simulink model "MIL4L3_SW6_V1_20220211"  (R2018b)
(part 32 of 52)

  Gain218/1 -> Data Type Conversion224/1, IMAPva_d_obj_status/1  "IMAPva_d_obj_status"
  Gain318/1 -> Data Type Conversion32/1, IMAPve_d_BCM_LowBeam_State/1
  SDFAva_g_obj_length/1 -> Gain214/1
  Gain67/1 -> Data Type Conversion96/1, IMAPve_d_TCU_AT_Failure/1
  Gain62/1 -> Data Type Conversion126/1, IMAPve_g_ESC_RR_WhlSpd/1
  Gain325/1 -> Data Type Conversion349/1, IMAPve_d_TBOX_LocalTimeS/1
  Gain63/1 -> Data Type Conversion127/1, IMAPve_d_ESC_FL_Wheel_Pulse/1
  Gain11/1 -> Data Type Conversion149/1, IMAPva_g_ORI_Obj_Width/1  "IMAPva_g_ORI_Obj_Width"
  Gain375/1 -> Data Type Conversion484/1, IMAPve_g_ORI_R1_Dxstart/1  "IMAPve_g_ORI_R1_Dxstart"
  ? -> Gain361/1
  Gain57/1 -> Data Type Conversion121/1, IMAPve_d_ESC_RL_WheelPulVal/1
  Data Type Conversion175/1 -> Terminator166/1  "ob_IMAPve_g_ORI_R0_C2"
  ? -> Gain369/1
  Data Type Conversion343/1 -> Terminator348/1  "ob_IMAPve_d_TBOX_LocalTimeM"
  Gain166/1 -> Data Type Conversion251/1, IMAPve_g_R0_C2/1  "IMAPve_g_R0_C2"
  Gain61/1 -> Data Type Conversion125/1, IMAPve_g_ESC_RL_WhlSpd/1
  Gain250/1 -> Data Type Conversion180/1, IMAPve_g_ORI_R0_VR/1  "IMAPve_g_ORI_R0_VR"
  Gain409/1 -> Data Type Conversion428/1, IMAPva_g_ORI_Obj_LAngleStdDev/1  "IMAPva_g_ORI_Obj_LAngleStdDev"
  Gain216/1 -> Data Type Conversion222/1, IMAPva_d_obj_class/1  "IMAPva_d_obj_class"
  Gain406/1 -> Data Type Conversion437/1, IMAPva_g_ORI_Obj_HeadingStdDev/1  "IMAPva_g_ORI_Obj_HeadingStdDev"
  Gain41/1 -> Data Type Conversion53/1, IMAPve_d_ACU_Driver_Belt/1
  Gain54/1 -> Data Type Conversion118/1, IMAPve_d_ESC_ABS_Active/1
  Gain60/1 -> Data Type Conversion124/1, IMAPve_g_ESC_FR_WhlSpd/1
  Gain211/1 -> Data Type Conversion413/1, IMAPve_d_MP5_APA_ModeSelect/1
  Data Type Conversion113/1 -> Terminator105/1  "ob_IMAPve_d_ESC_ESC_Active"
  Gain58/1 -> Data Type Conversion122/1, IMAPve_d_ESC_RR_WheelPulVal/1
  Gain441/1 -> IMAPve_d_ORI_FS_Fog/1, Data Type Conversion335/1  "IMAPve_d_ORI_FS_Fog"
  Data Type Conversion398/1 -> Terminator394/1  "ob_IMAPva_g_ORI_Obj_RelVelStdDev"
  SDFAve_g_ORI_L1_C1/1 -> Gain266/1
  Data Type Conversion194/1 -> Terminator185/1  "ob_IMAPve_d_LF_Radar_Status"
  Data Type Conversion318/1 -> Terminator309/1  "ob_IMAPve_d_MP5_DMS_UserAccount"
  Gain6/1 -> IMAPva_g_ORI_Obj_RelVel/1, Data Type Conversion144/1  "IMAPva_g_ORI_Obj_RelVel"
  Data Type Conversion250/1 -> Terminator241/1  "ob_IMAPve_g_R0_C1"
  Data Type Conversion170/1 -> Terminator161/1  "ob_IMAPve_g_ORI_L1_VR"
  Gain56/1 -> Data Type Conversion120/1, IMAPve_d_ESC_FR_WheelPulVal/1
  SDFAve_g_L1_VIEW_RANGE/1 -> Gain161/1
  Gain184/1 -> Data Type Conversion36/1, IMAPve_d_AEB_Switch/1
  Gain369/1 -> Data Type Conversion477/1, IMAPve_g_ORI_RoadedgeR0_C3/1  "IMAPve_g_ORI_RoadedgeR0_C3"
  Data Type Conversion253/1 -> Terminator244/1  "ob_IMAPve_g_R0_VR"
  SDFAve_g_ORI_R1_C0/1 -> Gain239/1
  Gain223/1 -> Data Type Conversion211/1, IMAPva_g_obj_acc_x/1  "IMAPva_g_obj_acc_x"
  SDFAve_g_R0_C3_BACK_COEF/1 -> Gain137/1
  Gain69/1 -> Data Type Conversion98/1, IMAPve_d_TCU_Gear_Engage/1
  Gain80/1 -> Data Type Conversion56/1, IMAPve_d_BCM_BrakeLamp_State/1
  Data Type Conversion157/1 -> Terminator148/1  "ob_IMAPve_g_ORI_L0_C0"
  Data Type Conversion211/1 -> Terminator202/1  "ob_IMAPva_g_obj_acc_x"
  ? -> Gain398/1
  Data Type Conversion283/1 -> Terminator274/1  "ob_IMAPve_g_L0_C1_Back"
  Gain230/1 -> Data Type Conversion195/1, IMAPve_d_RF_Radar_Status/1  "IMAPve_d_RF_Radar_Status"
  ? -> Gain358/1
  Gain44/1 -> Data Type Conversion88/1, IMAPve_d_TCU_Actual_Gear/1
  ? -> Gain375/1
  Gain52/1 -> Data Type Conversion116/1, IMAPve_d_ESC_VehSpd_Valid/1
  Data Type Conversion272/1 -> Terminator263/1  "ob_IMAPve_g_R1_C1"
  SDFAve_d_sen_sta_RF_radar/1 -> Gain230/1
  Gain109/1 -> Data Type Conversion201/1, IMAPve_d_TSR_Sign_Type/1  "IMAPve_d_TSR_Sign_Type"
  Data Type Conversion353/1 -> Terminator356/1  "ob_IMAPve_d_Outside_Temp"
  Gain143/1 -> Data Type Conversion282/1, IMAPve_g_L0_C0_Back/1  "IMAPve_g_L0_C0_Back"
  Gain55/1 -> Data Type Conversion119/1, IMAPve_d_ESC_FL_WheelPulVal/1
  Gain448/1 -> IMAPve_d_JA_Alert_Switch/1, Data Type Conversion24/1
  ? -> Gain377/1
  Gain33/1 -> Data Type Conversion81/1, IMAPve_g_EMS_MinTWhl/1
  Gain426/1 -> Data Type Conversion396/1, IMAPva_g_ORI_Obj_AbsAxStdDev/1  "IMAPva_g_ORI_Obj_AbsAxStdDev"
  Gain46/1 -> Data Type Conversion111/1, IMAPve_d_ESC_OFF/1
  Gain72/1 -> Data Type Conversion90/1, IMAPve_d_EMS_Gearbox_CtlAvail/1
  SWINve_y_MP5_DMS_SmokingMonitor/1 -> Gain301/1
  Gain144/1 -> Data Type Conversion283/1, IMAPve_g_L0_C1_Back/1  "IMAPve_g_L0_C1_Back"
  Data Type Conversion196/1 -> Terminator187/1  "ob_IMAPve_d_LR_Radar_Status"
  Gain145/1 -> Data Type Conversion284/1, IMAPve_g_L0_C2_Back/1  "IMAPve_g_L0_C2_Back"
  Gain32/1 -> Data Type Conversion80/1, IMAPve_g_EMS_MaxTWhl_Offset/1
  SDFAva_y_obj_class/1 -> Gain216/1
  Data Type Conversion421/1 -> Terminator402/1  "ob_IMAPva_g_ORI_Obj_ExistProb"
  Gain295/1 -> Data Type Conversion218/1, IMAPve_d_MP5_DMS_DelUserNum/1  "IMAPve_d_MP5_DMS_DelUserNum"
  Gain37/1 -> Data Type Conversion109/1, IMAPve_d_ESC_Brake_Effort/1
  SDFAve_g_L1_C2_BACK_COEF/1 -> Gain120/1
  Gain416/1 -> Data Type Conversion421/1, IMAPva_g_ORI_Obj_ExistProb/1  "IMAPva_g_ORI_Obj_ExistProb"
  Data Type Conversion67/1 -> Terminator58/1  "ob_IMAPve_d_SAS_Clb_State"
  Data Type Conversion122/1 -> Terminator114/1  "ob_IMAPve_d_ESC_RR_WheelPulVal"
  Gain39/1 -> Data Type Conversion110/1, IMAPve_d_ESC_Veh_Standstill/1
  Data Type Conversion221/1 -> Terminator212/1  "ob_IMAPve_d_MP5_DMS_Sensity"
  Gain432/1 -> IMAPva_g_ORI_Obj_AbsAy/1, Data Type Conversion393/1  "IMAPva_g_ORI_Obj_AbsAy"
  SDFAve_g_L1_BACK_RANGE/1 -> Gain122/1
  SDFAva_y_obj_MotionStatus/1 -> Gain206/1
  SWINve_y_MP5_DMS_SideViewMonitor/1 -> Gain299/1
  Gain35/1 -> Data Type Conversion77/1, IMAPve_g_EMS_Pot_WhlT_Min/1
  Gain246/1 -> Data Type Conversion176/1, IMAPve_g_ORI_R0_C1/1  "IMAPve_g_ORI_R0_C1"
  Data Type Conversion286/1 -> Terminator277/1  "ob_IMAPve_g_L0_Range_Back"
  Data Type Conversion344/1 -> Terminator349/1  "ob_IMAPve_d_TBOX_LocalTimeD"
  SWINve_y_MP5_DMS_UsingPhoneMonitor/1 -> Gain300/1
  ? -> Gain417/1
  Data Type Conversion204/1 -> Terminator195/1  "ob_IMAPve_d_Camera_Status"
  Data Type Conversion189/1 -> Terminator180/1  "ob_IMAPve_d_ORI_R1_LT"
  Gain42/1 -> array_transfer10/2(Left_Light), Data Type Conversion50/1, IMAPve_d_BCM_Left_Light/1
  ? -> Gain373/1
  Gain103/1 -> IMAPve_d_Camera_Status/1, Data Type Conversion204/1  "IMAPve_d_Camera_Status"
  Gain20/1 -> Data Type Conversion103/1, IMAPve_g_ESC_VehSpd/1
  Gain136/1 -> Data Type Conversion293/1, IMAPve_g_R0_C2_Back/1  "IMAPve_g_R0_C2_Back"
  Gain436/1 -> IMAPve_d_ORI_FS_FrozenWindshield0/1, Data Type Conversion389/1  "IMAPve_d_ORI_FS_FrozenWindshield0"
  Data Type Conversion406/1 -> Terminator335/1  "ob_IMAPve_d_BCM_LeftTurn_Switch"
  SDFAve_g_R1_C2_COEF/1 -> Gain152/1
  Data Type Conversion244/1 -> Terminator235/1  "ob_IMAPve_d_L0_Type"
  SDFAve_g_ORI_R1_VR/1 -> Gain242/1
  Gain238/1 -> Data Type Conversion186/1, IMAPve_g_ORI_R1_C1/1  "IMAPve_g_ORI_R1_C1"
  Gain262/1 -> Data Type Conversion162/1, IMAPve_g_ORI_L0_W/1  "IMAPve_g_ORI_L0_W"
  Data Type Conversion70/1 -> Terminator61/1  "ob_IMAPve_g_SW_Angle"
  SDFAve_y_R0_DETECT_QUALITY/1 -> Gain169/1
  Gain30/1 -> Data Type Conversion76/1, IMAPve_g_EMS_Pot_WhlT_Max/1
  Gain12/1 -> Data Type Conversion150/1, IMAPva_d_ORI_Obj_ID/1  "IMAPva_d_ORI_Obj_ID"
  Data Type Conversion249/1 -> Terminator240/1  "ob_IMAPve_g_R0_C0"
  Gain312/1 -> Data Type Conversion21/1, IMAPve_d_RCTA_Swtich/1
  Gain26/1 -> Data Type Conversion108/1, IMAPve_g_ESC_DySlope/1
  Data Type Conversion465/1 -> Terminator446/1  "ob_IMAPve_g_ORI_RoadedgeL0_DxEnd"
  ? -> Gain414/1
  Data Type Conversion42/1 -> Terminator33/1  "ob_IMAPve_d_BCM_Opening_State"
  Gain29/1 -> Data Type Conversion75/1, IMAPve_d_EMS_ACC_Status/1
  Data Type Conversion367/1 -> Terminator365/1  "ob_IMAPve_d_ESC_LatAcc_Valid"
  SWINve_y_MP5_DMS_DeleteUserNum/1 -> Gain295/1
  Data Type Conversion452/1 -> Terminator433/1  "ob_IMAPve_g_ORI_L0_TypeConf"
  Data Type Conversion165/1 -> Terminator156/1  "ob_IMAPve_g_ORI_L1_C2"
  Data Type Conversion167/1 -> Terminator158/1  "ob_IMAPve_g_ORI_L1_C0"
  Gain38/1 -> Data Type Conversion87/1, IMAPve_g_EMS_Engine_Speed/1
  Data Type Conversion453/1 -> Terminator434/1  "ob_IMAPve_g_ORI_R0_TypeConf"
  Gain65/1 -> Data Type Conversion129/1, IMAPve_d_ESC_RL_Wheel_Pulse/1
  Gain269/1 -> IMAPve_g_ORI_L0_C2/1, Data Type Conversion155/1  "IMAPve_g_ORI_L0_C2"
  SDFAve_d_ORI_Obj_Num/1 -> Gain2/1
  Data Type Conversion129/1 -> Terminator116/1  "ob_IMAPve_d_ESC_RL_Wheel_Pulse"
  Gain423/1 -> Data Type Conversion399/1, IMAPva_g_ORI_Obj_RelVelyStdDev/1  "IMAPva_g_ORI_Obj_RelVelyStdDev"
  SDFAva_g_obj_vel_x/1 -> Gain221/1
  SDFAve_d_ORI_L1_Type/1 -> Gain255/1
  SDFAva_g_ORI_Obj_AbsAy/1 -> Gain432/1
  Gain17/1 -> Data Type Conversion100/1, IMAPve_g_ESC_LatAcc/1
  Data Type Conversion145/1 -> Terminator136/1  "ob_IMAPva_g_ORI_Obj_LongDis"
  Gain372/1 -> Data Type Conversion480/1, IMAPve_d_ORI_RoadedgeR0_Type/1  "IMAPve_d_ORI_RoadedgeR0_Type"
  Gain36/1 -> Data Type Conversion86/1, IMAPve_g_EMS_Driver_Torque/1
  Data Type Conversion371/1 -> Terminator369/1  "ob_IMAPve_d_ESC_ABS_AlarmSig"
  Gain174/1 -> Data Type Conversion241/1, IMAPve_g_L0_C3/1  "IMAPve_g_L0_C3"
  Gain73/1 -> Data Type Conversion131/1, IMAPve_d_ESC_Brake_Failsafe/1
  Gain287/1 -> Data Type Conversion61/1, IMAPve_d_Time_System_Clock/1
  Gain234/1 -> Data Type Conversion199/1, IMAPve_d_Fusion_Time_Stamp/1  "IMAPve_d_Fusion_Time_Stamp"
  Gain48/1 -> IMAPve_d_BCM_Right_Light/1, Data Type Conversion51/1, array_transfer10/3(Right_Light)
  Gain40/1 -> Data Type Conversion52/1, IMAPve_d_BCM_Ignition_State/1
  ? -> Gain406/1
  Data Type Conversion147/1 -> Terminator138/1  "ob_IMAPva_g_ORI_Obj_LAngle"
  SDFAve_g_L0_VIEW_RANGE/1 -> Gain175/1
  Data Type Conversion99/1 -> Terminator90/1  "ob_IMAPve_d_TCU_Select_ATMode"
  Data Type Conversion187/1 -> Terminator178/1  "ob_IMAPve_g_ORI_R1_C0"
  Gain25/1 -> Data Type Conversion107/1, IMAPve_g_ESC_DySlope_Accuracy/1
  Data Type Conversion43/1 -> Terminator34/1  "ob_IMAPve_d_BCM_Trunk_State"
  Gain177/1 -> Data Type Conversion244/1, IMAPve_d_L0_Type/1  "IMAPve_d_L0_Type"
  SDFAva_g_ORI_Obj_RelVely/1 -> Gain444/1
  SDFAve_y_Radar_State/1 -> Gain102/1
  Data Type Conversion148/1 -> Terminator139/1  "ob_IMAPva_g_ORI_Obj_RAngle"
  Data Type Conversion350/1 -> Terminator353/1  "ob_IMAPve_d_TBOX_LocalTime_Valid"
  Gain4/1 -> Data Type Conversion142/1, IMAPva_d_ORI_Obj_Class/1  "IMAPva_d_ORI_Obj_Class"
  Data Type Conversion144/1 -> Terminator135/1  "ob_IMAPva_g_ORI_Obj_RelVel"
  Gain222/1 -> Data Type Conversion210/1, IMAPva_g_obj_vel_y/1  "IMAPva_g_obj_vel_y"
  ? -> Gain374/1
  Data Type Conversion156/1 -> Terminator147/1  "ob_IMAPve_g_ORI_L0_C1"
  SDFAve_d_sen_sta_LB_radar/1 -> Gain231/1
  Data Type Conversion160/1 -> Terminator151/1  "ob_IMAPve_g_ORI_L0_VR"
  Gain400/1 -> Data Type Conversion429/1, IMAPva_g_ORI_Obj_RAngleStdDev/1  "IMAPva_g_ORI_Obj_RAngleStdDev"
  Data Type Conversion238/1 -> Terminator229/1  "ob_IMAPve_g_L0_C0"
  Data Type Conversion159/1 -> Terminator150/1  "ob_IMAPve_d_ORI_L0_Type"
  Data Type Conversion275/1 -> Terminator266/1  "ob_IMAPve_g_R1_VR"
  Gain329/1 -> Data Type Conversion360/1, IMAPve_g_EPS_LKA_Current/1
  Data Type Conversion284/1 -> Terminator275/1  "ob_IMAPve_g_L0_C2_Back"
  Gain157/1 -> Data Type Conversion260/1, IMAPve_g_L1_C0/1  "IMAPve_g_L1_C0"
  Data Type Conversion140/1 -> Terminator131/1  "ob_IMAPve_d_ORI_Obj_Num"
  Gain9/1 -> IMAPva_g_ORI_Obj_LAngle/1, Data Type Conversion147/1  "ob_IMAPva_g_ORI_Obj_LAngle"
  Gain102/1 -> Data Type Conversion203/1, IMAPve_d_Radar_State/1  "IMAPve_d_Radar_Status"
  Gain224/1 -> Data Type Conversion212/1, IMAPva_g_obj_acc_y/1  "IMAPva_g_obj_acc_y"
  Gain88/1 -> Data Type Conversion74/1, IMAPve_d_EPS_Steer_Hold_State/1
  SDFAve_y_ISAPopupMessage/1 -> Gain450/1
  Data Type Conversion137/1 -> Terminator469/1  "ob_IMAPve_d_ISA_Popup_Message"
  Gain450/1 -> Data Type Conversion137/1, IMAPve_d_ISA_Popup_Message/1  "IMAPve_d_ISA_Popup_Message"
  Gain451/1 -> Data Type Conversion347/1, IMAPve_d_ISA_Sign_Type/1  "IMAPve_d_ISA_Sign_Type"
  SDFAve_y_ISASignType/1 -> Gain451/1
  Data Type Conversion347/1 -> Terminator470/1  "ob_IMAPve_d_ISA_Sign_Type"
  Gain452/1 -> Data Type Conversion488/1, IMAPve_d_ISA_Status/1  "IMAPve_d_ISA_Status"
  SDFAve_y_ISAStatus/1 -> Gain452/1
  Data Type Conversion488/1 -> Terminator471/1  "ob_IMAPve_d_ISA_Status"
  Gain105/1 -> Data Type Conversion198/1, IMAPve_d_Camera_State/1  "IMAPve_d_Camera_State"
  SDFAve_y_OperatingStatus/1 -> Gain105/1
  Data Type Conversion198/1 -> Terminator189/1  "ob_IMAPve_d_Camera_State"
  SDFAve_d_fusion_status/1 -> Gain233/1
  Gain233/1 -> Data Type Conversion7/1, IMAPve_d_Fusion_Status/1  "IMAPve_d_Fusion_Status"
  Data Type Conversion7/1 -> Terminator8/1  "ob_IMAPve_d_Fusion_Status"
  SWINve_y_LKA_main_switch/1 -> Switch/3
  Constant/1 -> Switch/1
  Constant1/1 -> Switch/2
  Gain3/1 -> IMAPve_d_LKA_Main_Switch/1, Data Type Conversion34/1
  Switch1/1 -> Gain183/1  "IMAPve_d_LKA_Mode"
  SWINve_y_LC_Mode/1 -> Switch1/3
  Constant2/1 -> Switch1/1
  Constant3/1 -> Switch1/2
  Switch2/1 -> Gain184/1  "IMAPve_d_AEB_Switch"
  SWINve_y_MP5_AEB_Activation_Config/1 -> Switch2/3
  Constant5/1 -> Switch2/2
  Constant4/1 -> Switch2/1
  Switch3/1 -> Gain185/1  "IMAPve_d_FCW_Switch"
  Constant6/1 -> Switch3/1
  Constant7/1 -> Switch3/2
  SWINve_y_IC_Fcw_Activation_Config/1 -> Switch3/3
  Switch4/1 -> Gain186/1  "IMAPve_d_FCW_Sensitivity"
  Constant9/1 -> Switch4/2
  Constant8/1 -> Switch4/1
  SWINve_y_IC_FCW_Sensitivity/1 -> Switch4/3
  Switch5/1 -> Gain187/1  "IMAPve_d_ISA_Switch"
  Constant11/1 -> Switch5/2
  Constant10/1 -> Switch5/1
  SWINve_y_GW_Mp5_ISA_Switch/1 -> Switch5/3
  Switch6/1 -> Gain188/1  "IMAPve_d_TSR_Switch"
  Constant13/1 -> Switch6/2
  Constant12/1 -> Switch6/1
  SWINve_y_GW_Mp5_TSR_Switch/1 -> Switch6/3
  Switch7/1 -> Gain304/1  "IMAPve_d_ISA_ISLC_Mode"
  Constant14/1 -> Switch7/1
  Constant15/1 -> Switch7/2
  SWINve_y_Mp5_ISAMode/1 -> Switch7/3
  Switch8/1 -> Gain305/1  "IMAPve_d_LDW_Warn_Mode"
  Constant16/1 -> Switch8/1
  Constant17/1 -> Switch8/2
  SWINve_y_Mp5_LDWWarningMode/1 -> Switch8/3
  Switch9/1 -> Gain306/1  "IMAPve_d_Speed_Limit"
  Constant20/1 -> Switch9/1
  Constant21/1 -> Switch9/2
  SWINve_y_MP5_ADASSpeedLimit/1 -> Switch9/3
  Switch10/1 -> Gain307/1  "IMAPve_d_ALC_TLC_Mode"
  Constant22/1 -> Switch10/1
  Constant23/1 -> Switch10/2
  SWINve_y_MP5_TLCModeSelection/1 -> Switch10/3
  Switch11/1 -> Gain308/1  "IMAPve_d_ESA_Switch"
  Constant24/1 -> Switch11/1
  Constant25/1 -> Switch11/2
  SWINve_y_MP5_ESASwitch/1 -> Switch11/3
  Switch12/1 -> Gain449/1  "IMAPve_d_ELK_Switch"
  Constant26/1 -> Switch12/1
  Constant27/1 -> Switch12/2
  SWINve_y_Mp5_ELKSwitch/1 -> Switch12/3
  Switch13/1 -> Gain309/1  "IMAPve_d_PEPS_RKE_Command"
  Constant29/1 -> Switch13/2
  Constant28/1 -> Switch13/1
  SWINve_y_PEPS_RKECommand/1 -> Switch13/3
  Switch14/1 -> Gain310/1  "IMAPve_d_BSD_LCW_Switch"
  Constant31/1 -> Switch14/2
  Constant30/1 -> Switch14/1
  SWINve_y_MP5_BSD_LCW_Activation/1 -> Switch14/3
  Switch15/1 -> Gain311/1  "IMAPve_d_FCTA_Switch"
  Constant32/1 -> Switch15/1
  Constant33/1 -> Switch15/2
  SWINve_y_MP5_FCTAActivation/1 -> Switch15/3
  Switch16/1 -> Gain312/1  "IMAPve_d_RCTA_Swtich"
  Constant35/1 -> Switch16/2
  Constant34/1 -> Switch16/1
  SWINve_y_MP5_RCTAActivation/1 -> Switch16/3
  Switch17/1 -> Gain313/1  "IMAPve_d_DOW_Switch"
  Constant37/1 -> Switch17/2
  Constant36/1 -> Switch17/1
  SWINve_y_MP5_DOWActivation/1 -> Switch17/3
  Switch18/1 -> Gain314/1  "IMAPve_d_JA_Brake_Switch"
  Constant38/1 -> Switch18/1
  Constant39/1 -> Switch18/2
  SWINve_y_MP5_JA_Modes/1 -> Switch18/3
  Switch19/1 -> Gain448/1  "IMAPve_d_JA_Alert_Switch"
  Constant41/1 -> Switch19/2
  Constant40/1 -> Switch19/1
  SWINve_y_MP5_JA_Alert_Switch/1 -> Switch19/3
  Switch20/1 -> Gain210/1  "IMAPve_d_MP5_Work_State"
  Constant42/1 -> Switch20/1
  Constant43/1 -> Switch20/2
  SWINve_y_MP5_WorkSt/1 -> Switch20/3
  Switch21/1 -> Gain211/1  "IMAPve_d_MP5_APA_ModeSelect"
  Constant45/1 -> Switch21/2
  Constant44/1 -> Switch21/1
  SWINve_y_MP5_APAModeSelect/1 -> Switch21/3
  Switch22/1 -> Gain212/1  "IMAPve_d_MP5_LanguageSet"
  Constant46/1 -> Switch22/1
  Constant47/1 -> Switch22/2
  SWINve_y_MP5_LanguageSet/1 -> Switch22/3
  Switch23/1 -> Gain215/1  "IMAPve_d_MP5_UPA_Switch"
  Constant49/1 -> Switch23/2
  Constant48/1 -> Switch23/1
  SWINve_y_MP5_UPASwitch/1 -> Switch23/3
  Switch24/1 -> Gain291/1  "IMAPve_d_MP5_FLK_Activation"
  Constant50/1 -> Switch24/1
  Constant51/1 -> Switch24/2
  SWINve_y_MP5_FLKActivation/1 -> Switch24/3
  Switch25/1 -> Gain292/1  "IMAPve_d_MP5_AutoPilot_Switch"
  Constant52/1 -> Switch25/1
  Constant53/1 -> Switch25/2
  SWINve_y_MP5_AutoPilotSwitch/1 -> Switch25/3
  SWINve_y_BCM_Status_Indicator/1 -> Gain282/1  "IMAPve_d_BCM_HazardLamp"
  Constant55/1 -> Switch26/2
  Constant54/1 -> Switch26/1
  Switch27/1 -> Gain42/1  "IMAPve_d_BCM_Left_Light"
  Constant57/1 -> Switch27/2
  Constant56/1 -> Switch27/1
  SWINve_y_BCM_LeftlightSt/1 -> Switch27/3
  Switch28/1 -> Gain48/1  "IMAPve_d_BCM_Right_Light"
  Constant59/1 -> Switch28/2
  Constant58/1 -> Switch28/1
  SWINve_y_BCM_RightlightSt/1 -> Switch28/3
  Switch29/1 -> Gain315/1  "IMAPve_d_ESC_BrakeLamp_Req"
  Constant60/1 -> Switch29/1
  Constant61/1 -> Switch29/2
  SWINve_y_ESC_BLRequest/1 -> Switch29/3
  Switch30/1 -> Gain53/1  "IMAPve_d_BCM_Trunk_State"
  Constant63/1 -> Switch30/2
  Constant62/1 -> Switch30/1
  SWINve_y_BCM_TrunkSt/1 -> Switch30/3
  Switch31/1 -> Gain76/1  "IMAPve_d_BCM_LF_Door_State"
  Constant65/1 -> Switch31/2
  Constant64/1 -> Switch31/1
  SWINve_y_BCM_LFDoorSwitchSt/1 -> Switch31/3
  Switch32/1 -> Gain279/1  "IMAPve_d_BCM_RF_Door_State"
  Constant66/1 -> Switch32/1
  Constant67/1 -> Switch32/2
  SWINve_y_BCM_RFDoorSwitchSt/1 -> Switch32/3
  Switch33/1 -> Gain289/1  "IMAPve_d_BCM_RR_Door_State"
  Constant69/1 -> Switch33/2
  Constant68/1 -> Switch33/1
  SWINve_y_BCM_RRDoorSwitchSt/1 -> Switch33/3
  Switch34/1 -> Gain353/1  "IMAPve_d_BCM_LR_Door_State"
  Constant70/1 -> Switch34/1
  Constant71/1 -> Switch34/2
  SWINve_y_BCM_LRDoorSwitchSt/1 -> Switch34/3
  Switch35/1 -> Gain27/1  "IMAPve_d_SCC_Left_SwitchSig"
  Constant73/1 -> Switch35/2
  Constant72/1 -> Switch35/1
  SWINve_y_GW_SCC_LeftSteeringWheelSwitch/1 -> Switch35/3
  Switch36/1 -> Gain28/1  "IMAPve_d_SCC_Right_SwitchSig"
  Constant74/1 -> Switch36/1
  Constant75/1 -> Switch36/2
  SWINve_y_GW_SCC_RightSteeringWheelSwitch/1 -> Switch36/3
  Switch37/1 -> Gain316/1  "IMAPve_d_PEPS_Door_Lock_Req"
  Constant76/1 -> Switch37/1
  Constant77/1 -> Switch37/2
  SWINve_y_PEPS_DoorLockReq/1 -> Switch37/3
  Switch38/1 -> Gain317/1  "IMAPve_d_BCM_Door_Lock_State"
  Constant79/1 -> Switch38/2
  Constant78/1 -> Switch38/1
  SWINve_y_BCM_DoorLockSt/1 -> Switch38/3
  Switch39/1 -> Gain40/1  "IMAPve_d_BCM_Ignition_State"
  Constant80/1 -> Switch39/1
  Constant81/1 -> Switch39/2
  SWINve_y_GW_BCM_SEV_main_state/1 -> Switch39/3
  Switch40/1 -> Gain41/1  "IMAPve_d_ACU_Driver_Belt"
  Constant83/1 -> Switch40/2
  Constant82/1 -> Switch40/1
  SWINve_y_IC_seat_bealt_driver_state/1 -> Switch40/3
  Switch41/1 -> Gain78/1  "IMAPve_d_BCM_FrontWiper_State"
  Constant85/1 -> Switch41/2
  Constant84/1 -> Switch41/1
  SWINve_y_BCM_State_Front_Wiper/1 -> Switch41/3
  Switch42/1 -> Gain79/1  "IMAPve_d_BCM_CHMSL_Status"
  Switch43/1 -> Gain80/1  "IMAPve_d_BCM_BrakeLamp_State"
  Constant87/1 -> Switch42/2
  Constant86/1 -> Switch42/1
  SWINve_y_BCM_CHMSLStatus/1 -> Switch42/3
  Constant89/1 -> Switch43/2
  Constant88/1 -> Switch43/1
  SWINve_y_BCM_BrakeLampStatus/1 -> Switch43/3
  Switch44/1 -> Gain75/1  "IMAPve_d_ACU_Passenger_Belt"
  Switch45/1 -> Gain318/1  "IMAPve_d_BCM_LowBeam_State"
  Switch46/1 -> Gain85/1  "IMAPve_d_BCM_HighBeam_State"
  Constant91/1 -> Switch44/2
  Constant90/1 -> Switch44/1
  SWINve_y_IC_passengerBeltSwitchSig/1 -> Switch44/3
  Constant92/1 -> Switch45/1
  Constant93/1 -> Switch45/2
  SWINve_y_BCM_LowBeamStatus/1 -> Switch45/3
  Constant94/1 -> Switch46/1
  Constant95/1 -> Switch46/2
  SWINve_y_High_beam_state/1 -> Switch46/3
  Switch47/1 -> Gain319/1  "IMAPve_g_BCM_Battery_Voltage"
  Constant96/1 -> Switch47/1
  Constant97/1 -> Switch47/2
  SWINve_g_BCM_BattVolt/1 -> Switch47/3
  Switch48/1 -> Gain320/1  "IMAPve_d_TBOX_LocalTimeY"
  Constant99/1 -> Switch48/2
  Constant98/1 -> Switch48/1
  SWINve_d_TBOX_LocalTimeYear/1 -> Switch48/3
  Switch49/1 -> Gain321/1  "IMAPve_d_TBOX_LocalTimeM"
  Constant101/1 -> Switch49/2
  Constant100/1 -> Switch49/1
  SWINve_y_TBOX_LocalTimeMonth/1 -> Switch49/3
  Switch50/1 -> Gain322/1  "IMAPve_d_TBOX_LocalTimeD"
  Constant103/1 -> Switch50/2
  Constant102/1 -> Switch50/1
  SWINve_y_TBOX_LocalTimeDate/1 -> Switch50/3
  Switch51/1 -> Gain323/1  "IMAPve_d_TBOX_LocalTimeH"
  Constant105/1 -> Switch51/2
  Constant104/1 -> Switch51/1
  SWINve_y_TBOX_LocalTimeHour/1 -> Switch51/3
  Switch52/1 -> Gain324/1  "IMAPve_d_TBOX_LocalTimeMin"
  Constant106/1 -> Switch52/1
  Constant107/1 -> Switch52/2
  SWINve_y_TBOX_LocalTimeMinute/1 -> Switch52/3
  Switch53/1 -> Gain325/1  "IMAPve_d_TBOX_LocalTimeS"
  Switch54/1 -> Gain326/1  "IMAPve_d_TBOX_LocalTime_Valid"
  Constant109/1 -> Switch53/2
  Constant108/1 -> Switch53/1
  SWINve_y_TBOX_LocalTimeSecond/1 -> Switch53/3
  Constant111/1 -> Switch54/2
  Constant110/1 -> Switch54/1
  SWINve_y_TBOX_LocalTimeValid/1 -> Switch54/3
  Switch55/1 -> Gain287/1  "IMAPve_d_Time_System_Clock"
  Constant112/1 -> Switch55/1
  Constant113/1 -> Switch55/2
  System_Clock/1 -> Switch55/3
  Switch56/1 -> Gain100/1  "IMAPve_g_GW_IC_Odometer"
  Constant115/1 -> Switch56/2
  Constant114/1 -> Switch56/1
  SWINve_g_number_of_kilometer/1 -> Switch56/3
  Switch57/1 -> Gain327/1  "IMAPve_d_Outside_Temp"
  Constant117/1 -> Switch57/2
  Constant116/1 -> Switch57/1
  SWINve_g_AC_AmbTemp/1 -> Switch57/3
  Switch58/1 -> Gain99/1  "IMAPve_d_ACU_RearLeft_Belt"
  Constant119/1 -> Switch58/2
  Constant118/1 -> Switch58/1
  SWINve_y_ACU_RearLeftBeltSwitchSig/1 -> Switch58/3
  Switch59/1 -> Gain192/1  "IMAPve_d_ACU_RearMiddle_Belt"
  Constant121/1 -> Switch59/2
  Constant120/1 -> Switch59/1
  SWINve_y_ACU_RearMiddleBeltSwitchSig/1 -> Switch59/3
  Switch60/1 -> Gain193/1  "IMAPve_d_ACU_RearRight_Belt"
  Constant123/1 -> Switch60/2
  Constant122/1 -> Switch60/1
  SWINve_y_ACU_RearRightBeltSwitchSig/1 -> Switch60/3
  Switch61/1 -> Gain202/1  "IMAPve_d_BCM_LeftTurn_Switch"
  Constant124/1 -> Switch61/1
  Constant125/1 -> Switch61/2
  SWINve_y_BCM_LeftTurnSwitchSt/1 -> Switch61/3
  Switch62/1 -> Gain207/1  "IMAPve_d_BCM_RightTurn_Switch"
  Constant127/1 -> Switch62/2
  Constant126/1 -> Switch62/1
  SWINve_y_BCM_RightTurnSwitchSt/1 -> Switch62/3
  Switch63/1 -> Gain208/1  "IMAPve_d_BCM_FrontWiper_Switch"
  Switch64/1 -> Gain209/1  "IMAPve_d_BCM_IHBC_Enabled"
  Constant129/1 -> Switch63/2
  Constant128/1 -> Switch63/1
  SWINve_y_BCM_FrontWiperSwitchSt/1 -> Switch63/3
  Constant130/1 -> Switch64/1
  Constant131/1 -> Switch64/2
  SWINve_y_BCM_IHBC_Function_Enabled/1 -> Switch64/3
  Switch65/1 -> Gain189/1  "IMAPve_d_EPS_LKA_State"
  Constant133/1 -> Switch65/2
  Constant132/1 -> Switch65/1
  SWINve_y_State_of_EPS_for_LKA_function/1 -> Switch65/3
  Switch66/1 -> Gain190/1  "IMAPve_g_EPS_SW_Trq"
  Constant134/1 -> Switch66/1
  Constant135/1 -> Switch66/2
  SWINve_g_Steering_wheel_torque/1 -> Switch66/3
  Switch67/1 -> Gain328/1  "IMAPve_d_EPS_Trq_State"
  Constant137/1 -> Switch67/2
  Constant136/1 -> Switch67/1
  SWINve_y_EPS_SteeringTorqueSensorSt/1 -> Switch67/3
  Switch68/1 -> Gain15/1  "IMAPve_d_SAS_Clb_State"
  Constant138/1 -> Switch68/1
  Constant139/1 -> Switch68/2
  SWINve_y_SWS_calibration/1 -> Switch68/3
  Switch69/1 -> Gain16/1  "IMAPve_d_SAS_Trim_State"
  Constant140/1 -> Switch69/1
  Constant141/1 -> Switch69/2
  SWINve_y_SWS_trim/1 -> Switch69/3
  Switch70/1 -> Gain280/1  "IMAPve_d_EPS_TrqLim_State"
  Constant142/1 -> Switch70/1
  Constant143/1 -> Switch70/2
  SWINve_y_Torque_limitation_if_DAE_limit/1 -> Switch70/3
  Switch71/1 -> Gain329/1  "IMAPve_g_EPS_LKA_Current"
  Constant144/1 -> Switch71/1
  Constant145/1 -> Switch71/2
  SWINve_g_EPS_LKACurrentOverlay/1 -> Switch71/3
  Switch72/1 -> Switch174/1, Gain281/1  "IMAPve_g_SW_Angle"
  Constant146/1 -> Switch72/1
  Constant147/1 -> Switch72/2
  SWINve_g_Steering_wheel_angle/1 -> Switch72/3
  Switch73/1 -> Gain24/1  "IMAPve_g_SW_Angle_Speed"
  Constant148/1 -> Switch73/1
  Constant149/1 -> Switch73/2
  SWINve_g_Steering_wheel_rotation_speed/1 -> Switch73/3
  Switch74/1 -> Gain43/1  "IMAPve_d_SWS_Failure_Status"
  Constant150/1 -> Switch74/1
  Constant151/1 -> Switch74/2
  SWINve_y_Internal_SWS_status/1 -> Switch74/3
  Switch75/1 -> Gain88/1  "IMAPve_d_EPS_Steer_Hold_State"
  Constant152/1 -> Switch75/1
  Constant153/1 -> Switch75/2
  SWINve_y_State_indicating_steer_or_not/1 -> Switch75/3
  Switch76/1 -> Gain330/1  "IMAPve_d_EPS_Warning_State"
  Constant154/1 -> Switch76/1
  Constant155/1 -> Switch76/2
  SWINve_y_EPS_WarningLampSt/1 -> Switch76/3
  Switch77/1 -> Gain331/1  "IMAPve_g_EPS_PowerCon"
  Constant156/1 -> Switch77/1
  Constant157/1 -> Switch77/2
  SWINve_g_EPS_ElectPowerConsumption/1 -> Switch77/3
  Switch78/1 -> Gain94/1  "IMAPve_d_EPS_SteeringAngle_Flag"
  Constant158/1 -> Switch78/1
  Constant159/1 -> Switch78/2
  SWINve_y_EPS_SteeringAngle_Flag/1 -> Switch78/3
  Switch79/1 -> Switch174/3  "IMAPve_g_EPS_SteeringAngle"
  Constant160/1 -> Switch79/1
  Constant161/1 -> Switch79/2
  SWINve_g_EPS_SteeringAngle/1 -> Switch79/3
  Switch80/1 -> Gain96/1  "IMAPve_d_EPS_Driver_Override"
  Constant162/1 -> Switch80/1
  Constant163/1 -> Switch80/2
  SWINve_y_EPS_DriverOverride/1 -> Switch80/3
  Switch81/1 -> Gain97/1  "IMAPve_d_EPS_Driver_Active_ESA"
  Constant164/1 -> Switch81/1
  Constant165/1 -> Switch81/2
  SWINve_y_EPS_DriverInitializedESA/1 -> Switch81/3
  Switch82/1 -> Gain98/1  "IMAPve_d_EPS_ESA_State"
  Constant166/1 -> Switch82/1
  Constant167/1 -> Switch82/2
  SWINve_y_EPS_ESAState/1 -> Switch82/3
  Switch83/1 -> Gain29/1  "IMAPve_d_EMS_ACC_Status"
  Constant169/1 -> Switch83/2
  Constant168/1 -> Switch83/1
  SWINve_y_GW_EMS_EMS_Status_ACC/1 -> Switch83/3
  Switch84/1 -> Gain30/1  "IMAPve_g_EMS_Pot_WhlT_Max"
  Constant171/1 -> Switch84/2
  Constant170/1 -> Switch84/1
  SWINve_g_GW_EMS_Pot_WhlTrq_Max/1 -> Switch84/3
  Switch85/1 -> Gain35/1  "IMAPve_g_EMS_Pot_WhlT_Min"
  Constant173/1 -> Switch85/2
  Constant172/1 -> Switch85/1
  SWINve_g_GW_EMS_Pot_WhlTrq_Min/1 -> Switch85/3
  Switch86/1 -> Gain278/1  "IMAPve_g_EMS_RealPedal"
  Constant175/1 -> Switch86/2
  Constant174/1 -> Switch86/1
  SWINve_g_EMS_Acceleration_pedal_position/1 -> Switch86/3
  Switch87/1 -> Gain31/1  "IMAPve_g_EMS_MaxTWhl"
  Constant177/1 -> Switch87/2
  Constant176/1 -> Switch87/1
  SWINve_g_EMS_WhlTrq_max/1 -> Switch87/3
  Switch88/1 -> Gain32/1  "IMAPve_g_EMS_MaxTWhl_Offset"
  Constant179/1 -> Switch88/2
  Constant178/1 -> Switch88/1
  SWINve_g_EMS_WhlTrq_max_offset/1 -> Switch88/3
  Switch89/1 -> Gain33/1  "IMAPve_g_EMS_MinTWhl"
  Constant181/1 -> Switch89/2
  Constant180/1 -> Switch89/1
  SWINve_g_EMS_WhlTrq_min/1 -> Switch89/3
  Switch90/1 -> Gain34/1  "IMAPve_g_EMS_MinTWhl_Offset"
  Constant183/1 -> Switch90/2
  Constant182/1 -> Switch90/1
  SWINve_g_EMS_WhlTrq_min_offset/1 -> Switch90/3
  Switch91/1 -> Gain283/1  "IMAPve_g_EMS_Actual_FlwT"
  Constant185/1 -> Switch91/2
  Constant184/1 -> Switch91/1
  SWINve_g_EMS_Actual_torque/1 -> Switch91/3
  Switch92/1 -> Gain332/1  "IMAPve_g_EMS_Actual_IndT"
  Constant187/1 -> Switch92/2
  Constant186/1 -> Switch92/1
  SWINve_g_EMS_EngActualIndTorque/1 -> Switch92/3
  Switch93/1 -> Gain284/1  "IMAPve_g_EMS_Realize_TWhl"
  Constant189/1 -> Switch93/2
  Constant188/1 -> Switch93/1
  SWINve_g_EMS_Actual_whlTrq/1 -> Switch93/3
  Switch94/1 -> Gain285/1  "IMAPve_g_EMS_ACC_VirtualPedal"
  Constant191/1 -> Switch94/2
  Constant190/1 -> Switch94/1
  SWINve_g_EMS_Driver_request/1 -> Switch94/3
  Switch95/1 -> Gain333/1  "IMAPve_d_EMS_AccPedal_Fault"
  Constant193/1 -> Switch95/2
  Constant192/1 -> Switch95/1
  SWINve_y_EMS_AccPedalFaultBit/1 -> Switch95/3
  Switch96/1 -> Gain36/1  "IMAPve_g_EMS_Driver_Torque"
  Constant195/1 -> Switch96/2
  Constant194/1 -> Switch96/1
  SWINve_g_EMS_Driver_wheel_torque/1 -> Switch96/3
  Switch97/1 -> Gain38/1  "IMAPve_g_EMS_Engine_Speed"
  Constant197/1 -> Switch97/2
  Constant196/1 -> Switch97/1
  SWINve_g_EMS_Engine_RPM/1 -> Switch97/3
  Switch98/1 -> Gain44/1  "IMAPve_d_TCU_Actual_Gear"
  Constant199/1 -> Switch98/2
  Constant198/1 -> Switch98/1
  SWINve_y_TCU_Gear_lever_position/1 -> Switch98/3
  Switch99/1 -> Gain45/1  "IMAPve_d_TCU_Target_Gear"
  Constant200/1 -> Switch99/1
  Constant201/1 -> Switch99/2
  SWINve_y_TCU_AGB_Target_position/1 -> Switch99/3
  Switch100/1 -> Gain334/1  "IMAPve_d_TCU_PRND_State"
  Constant203/1 -> Switch100/2
  Constant202/1 -> Switch100/1
  SWINve_y_TCU_PRNDLStatus/1 -> Switch100/3
  Switch101/1 -> Gain67/1  "IMAPve_d_TCU_AT_Failure"
  Constant205/1 -> Switch101/2
  Constant204/1 -> Switch101/1
  SWINve_y_TCU_ATFailure/1 -> Switch101/3
  Switch102/1 -> Gain335/1  "IMAPve_d_TCU_Shift_Valid"
  Constant207/1 -> Switch102/2
  Constant206/1 -> Switch102/1
  SWINve_y_TCU_ShiftLeverPosValidFlag/1 -> Switch102/3
  Switch103/1 -> Gain68/1  "IMAPve_d_TCU_DCT_Clutch_State"
  Constant209/1 -> Switch103/2
  Constant208/1 -> Switch103/1
  SWINve_y_TCU_DCTClutchStatus/1 -> Switch103/3
  Switch104/1 -> Gain69/1  "IMAPve_d_TCU_Gear_Engage"
  Constant211/1 -> Switch104/2
  Constant210/1 -> Switch104/1
  SWINve_y_TCU_GearEngagement/1 -> Switch104/3
  Switch105/1 -> Gain70/1  "IMAPve_d_TCU_Select_ATMode"
  Constant213/1 -> Switch105/2
  Constant212/1 -> Switch105/1
  SWINve_y_TCU_PROGRAMME_ACC/1 -> Switch105/3
  Switch106/1 -> Gain71/1  "IMAPve_d_EMS_Engine_Status"
  Constant215/1 -> Switch106/2
  Constant214/1 -> Switch106/1
  SWINve_y_EMS_Engine_state/1 -> Switch106/3
  Switch107/1 -> Gain72/1  "IMAPve_d_EMS_Gearbox_CtlAvail"
  Constant217/1 -> Switch107/2
  Constant216/1 -> Switch107/1
  SWINve_y_EMS_GearBox_ACC_Ctl_Available/1 -> Switch107/3
  Switch108/1 -> Gain77/1  "IMAPve_d_EMS_ACC_Effective"
  Constant219/1 -> Switch108/2
  Constant218/1 -> Switch108/1
  SWINve_y_EMS_ACC_Effecitive_EMS/1 -> Switch108/3
  Switch109/1 -> Gain81/1  "IMAPve_d_EMS_ACC_CtlAvail"
  Constant221/1 -> Switch109/2
  Constant220/1 -> Switch109/1
  SWINve_y_EMS_ACCcontrol_Available/1 -> Switch109/3
  Switch110/1 -> Gain82/1  "IMAPve_d_EMS_ACC_Inhibited"
  Constant223/1 -> Switch110/2
  Constant222/1 -> Switch110/1
  SWINve_y_GW_EMS_ACC_Ihibited_By_Engine/1 -> Switch110/3
  Switch111/1 -> Gain83/1  "IMAPve_d_EMS_Brake_Pedal"
  Constant225/1 -> Switch111/2
  Constant224/1 -> Switch111/1
  SWINve_y_Brake_secondary_contact/1 -> Switch111/3
  Switch112/1 -> Gain194/1  "IMAPve_d_EMS_PowertrainCtl_State"
  Constant227/1 -> Switch112/2
  Constant226/1 -> Switch112/1
  SWINve_y_EMS_PowertrainControlSt/1 -> Switch112/3
  Switch113/1 -> Gain201/1  "IMAPve_d_TCU_TCU_Available"
  Constant229/1 -> Switch113/2
  Constant228/1 -> Switch113/1
  SWINve_y_TCU_TCUAvailable/1 -> Switch113/3
  Switch114/1 -> Gain17/1  "IMAPve_g_ESC_LatAcc"
  Constant231/1 -> Switch114/2
  Constant230/1 -> Switch114/1
  SWINve_g_Lateral_acceleration/1 -> Switch114/3
  Switch115/1 -> Gain352/1  "IMAPve_d_ESC_LatAcc_Valid"
  Constant233/1 -> Switch115/2
  Constant232/1 -> Switch115/1
  SWINve_y_ESC_LateralAccelarationValidity/1 -> Switch115/3
  Switch116/1 -> Gain18/1  "IMAPve_g_ESC_YawRate"
  Constant235/1 -> Switch116/2
  Constant234/1 -> Switch116/1
  SWINve_g_Yaw_speed/1 -> Switch116/3
  Switch117/1 -> Gain351/1  "IMAPve_d_ESC_YawRate_Valid"
  Constant237/1 -> Switch117/2
  Constant236/1 -> Switch117/1
  SWINve_y_ESC_YawrateValidity/1 -> Switch117/3
  Switch118/1 -> Gain19/1  "IMAPve_g_ESC_UnYawRate"
  Constant239/1 -> Switch118/2
  Constant238/1 -> Switch118/1
  SWINve_g_YawRate_Raw/1 -> Switch118/3
  Switch119/1 -> Gain20/1  "IMAPve_g_ESC_VehSpd"
  Constant241/1 -> Switch119/2
  Constant240/1 -> Switch119/1
  SWINve_g_Vehicle_speed_of_wheelsensor/1 -> Switch119/3
  Switch120/1 -> Gain21/1  "IMAPve_g_ESC_LonAcc"
  Constant243/1 -> Switch120/2
  Constant242/1 -> Switch120/1
  SWINve_g_ACCEL_LONGI_CALIB/1 -> Switch120/3
  Switch121/1 -> Gain350/1  "IMAPve_d_ESC_LonAcc_Valid"
  Constant245/1 -> Switch121/2
  Constant244/1 -> Switch121/1
  SWINve_y_ESC_LongitudinalAccelerationValidity/1 -> Switch121/3
  Switch122/1 -> Gain22/1  "IMAPve_g_ESC_Brake_Press"
  Constant247/1 -> Switch122/2
  Constant246/1 -> Switch122/1
  SWINve_g_TMC_pressure/1 -> Switch122/3
  Switch123/1 -> Gain23/1  "IMAPve_g_ESC_Static_Slope"
  Constant249/1 -> Switch123/2
  Constant248/1 -> Switch123/1
  SWINve_g_Static_slope/1 -> Switch123/3
  Switch124/1 -> Gain25/1  "IMAPve_g_ESC_DySlope_Accuracy"
  Constant251/1 -> Switch124/2
  Constant250/1 -> Switch124/1
  SWINve_y_Dynamic_slope_accuracy/1 -> Switch124/3
  Switch125/1 -> Gain26/1  "IMAPve_g_ESC_DySlope"
  Constant253/1 -> Switch125/2
  Constant252/1 -> Switch125/1
  SWINve_y_Dynamic_slope/1 -> Switch125/3
  Switch126/1 -> Gain37/1  "IMAPve_d_ESC_Brake_Effort"
  Constant255/1 -> Switch126/2
  Constant254/1 -> Switch126/1
  SWINve_y_Braking_effort/1 -> Switch126/3
  Switch127/1 -> Gain39/1  "IMAPve_d_ESC_Veh_Standstill"
  Constant257/1 -> Switch127/2
  Constant256/1 -> Switch127/1
  SWINve_y_Vehicle_detected_as_stationary/1 -> Switch127/3
  Switch128/1 -> Gain46/1  "IMAPve_d_ESC_OFF"
  Constant259/1 -> Switch128/2
  Constant258/1 -> Switch128/1
  SWINve_y_ASR_ESP_disconnected/1 -> Switch128/3
  Switch129/1 -> Gain47/1  "IMAPve_d_ESC_AlarmSig"
  Constant261/1 -> Switch129/2
  Constant260/1 -> Switch129/1
  SWINve_y_Request_to_light_fault_lamp/1 -> Switch129/3
  Switch130/1 -> Gain49/1  "IMAPve_d_ESC_ESC_Active"
  Constant263/1 -> Switch130/2
  Constant262/1 -> Switch130/1
  SWINve_y_ESP_in_regulation/1 -> Switch130/3
  Switch131/1 -> Gain50/1  "IMAPve_d_ESC_MSR_Active"
  Constant265/1 -> Switch131/2
  Constant264/1 -> Switch131/1
  SWINve_y_MSR_in_regulation/1 -> Switch131/3
  Switch132/1 -> Gain51/1  "IMAPve_d_ESC_TCS_Active"
  Constant267/1 -> Switch132/2
  Constant266/1 -> Switch132/1
  SWINve_y_ASR_in_regulation/1 -> Switch132/3
  Switch133/1 -> Gain52/1  "IMAPve_d_ESC_VehSpd_Valid"
  Constant269/1 -> Switch133/2
  Constant268/1 -> Switch133/1
  SWINve_y_Vehiclespd_unavailability_flag/1 -> Switch133/3
  Switch134/1 -> Gain54/1  "IMAPve_d_ESC_ABS_Active"
  Constant271/1 -> Switch134/2
  Constant270/1 -> Switch134/1
  SWINve_y_ABS_in_regulation/1 -> Switch134/3
  Switch135/1 -> Gain348/1  "IMAPve_d_ESC_ABS_Valid"
  Constant273/1 -> Switch135/2
  Constant272/1 -> Switch135/1
  SWINve_y_ESC_ABSValidity/1 -> Switch135/3
  Switch136/1 -> Gain349/1  "IMAPve_d_ESC_ABS_AlarmSig"
  Constant275/1 -> Switch136/2
  Constant274/1 -> Switch136/1
  SWINve_y_ESC_ABSAlarmSig/1 -> Switch136/3
  Switch137/1 -> Gain55/1  "IMAPve_d_ESC_FL_WheelPulVal"
  Constant277/1 -> Switch137/2
  Constant276/1 -> Switch137/1
  SWINve_y_Front_Left_pulse_malfunction/1 -> Switch137/3
  Switch138/1 -> Gain56/1  "IMAPve_d_ESC_FR_WheelPulVal"
  Constant279/1 -> Switch138/2
  Constant278/1 -> Switch138/1
  SWINve_y_Front_right_pulse_malfunction/1 -> Switch138/3
  Switch139/1 -> Gain57/1  "IMAPve_d_ESC_RL_WheelPulVal"
  Constant281/1 -> Switch139/2
  Constant280/1 -> Switch139/1
  SWINve_y_Rear_Left_pulse_malfunction/1 -> Switch139/3
  Switch140/1 -> Gain58/1  "IMAPve_d_ESC_RR_WheelPulVal"
  Constant283/1 -> Switch140/2
  Constant282/1 -> Switch140/1
  SWINve_y_Rear_Right_pulse_malfunction/1 -> Switch140/3
  Switch141/1 -> Gain59/1  "IMAPve_g_ESC_FL_WhlSpd"
  Constant285/1 -> Switch141/2
  Constant284/1 -> Switch141/1
  SWINve_g_No_filtered_front_left_speed/1 -> Switch141/3
  Switch142/1 -> Gain347/1  "IMAPve_d_ESC_FL_WhlSpd_Fault"
  Constant287/1 -> Switch142/2
  Constant286/1 -> Switch142/1
  SWINve_y_ESC_FLWHeelSpdFaultSignal/1 -> Switch142/3
  Switch143/1 -> Gain60/1  "IMAPve_g_ESC_FR_WhlSpd"
  Constant289/1 -> Switch143/2
  Constant288/1 -> Switch143/1
  SWINve_g_No_filtered_front_right_speed/1 -> Switch143/3
  Switch144/1 -> Gain346/1  "IMAPve_d_ESC_FR_WhlSpd_Fault"
  Constant291/1 -> Switch144/2
  Constant290/1 -> Switch144/1
  SWINve_y_ESC_FRWHeelSpdFaultSignal/1 -> Switch144/3
  Switch145/1 -> Gain61/1  "IMAPve_g_ESC_RL_WhlSpd"
  Constant292/1 -> Switch145/1
  Constant293/1 -> Switch145/2
  SWINve_g_No_filtered_rear_left_speed/1 -> Switch145/3
  Switch146/1 -> Gain286/1  "IMAPve_d_ESC_RL_WhlSpd_Fault"
  Constant295/1 -> Switch146/2
  Constant294/1 -> Switch146/1
  SWINve_y_ESC_RLWHeelSpdFaultSignal/1 -> Switch146/3
  Switch147/1 -> Gain62/1  "IMAPve_g_ESC_RR_WhlSpd"
  Constant297/1 -> Switch147/2
  Constant296/1 -> Switch147/1
  SWINve_g_No_filtered_rear_rignt_speed/1 -> Switch147/3
  Switch148/1 -> Gain74/1  "IMAPve_d_ESC_RR_WhlSpd_Fault"
  Constant299/1 -> Switch148/2
  Constant298/1 -> Switch148/1
  SWINve_y_ESC_RRWHeelSpdFaultSignal/1 -> Switch148/3
  Switch149/1 -> Gain63/1  "IMAPve_d_ESC_FL_Wheel_Pulse"
  Constant301/1 -> Switch149/2
  Constant300/1 -> Switch149/1
  SWINve_g_Pulse_counter_front_left_wheel/1 -> Switch149/3
  Switch150/1 -> Gain64/1  "IMAPve_d_ESC_FR_Wheel_Pulse"
  Constant303/1 -> Switch150/2
  Constant302/1 -> Switch150/1
  SWINve_g_Pulse_counter_front_right_wheel/1 -> Switch150/3
  Switch151/1 -> Gain65/1  "IMAPve_d_ESC_RL_Wheel_Pulse"
  Constant305/1 -> Switch151/2
  Constant304/1 -> Switch151/1
  SWINve_g_Pulse_counter_rearleft_wheel/1 -> Switch151/3
  Switch152/1 -> Gain66/1  "IMAPve_d_ESC_RR_Wheel_Pulse"
  Constant307/1 -> Switch152/2
  Constant306/1 -> Switch152/1
  SWINve_g_Pulse_counter_rearright_wheel/1 -> Switch152/3
  Switch153/1 -> Gain73/1  "IMAPve_d_ESC_Brake_Failsafe"
  Constant309/1 -> Switch153/2
  Constant308/1 -> Switch153/1
  SWINve_y_Message_from_ESC_informing/1 -> Switch153/3
  Switch154/1 -> Gain342/1  "IMAPve_d_ESC_AEB_Available"
  Constant311/1 -> Switch154/2
  Constant310/1 -> Switch154/1
  SWINve_y_ESC_AEBAvailable/1 -> Switch154/3
  Switch155/1 -> Gain343/1  "IMAPve_d_ESC_AEB_Active"
  Constant313/1 -> Switch155/2
  Constant312/1 -> Switch155/1
  SWINve_y_ESC_AEBActive/1 -> Switch155/3
  Switch156/1 -> Gain344/1  "IMAPve_d_ESC_ACC_Available"
  Constant315/1 -> Switch156/2
  Constant314/1 -> Switch156/1
  SWINve_y_ESC_ACCAvailable/1 -> Switch156/3
  Switch157/1 -> Gain345/1  "IMAPve_d_ESC_ACC_Active"
  Constant317/1 -> Switch157/2
  Constant316/1 -> Switch157/1
  SWINve_y_ESC_ACCActive/1 -> Switch157/3
  Switch158/1 -> Gain290/1  "IMAPve_d_EPB_Status"
  Constant319/1 -> Switch158/2
  Constant318/1 -> Switch158/1
  SWINve_y_Park_brake_function_status/1 -> Switch158/3
  Switch159/1 -> Gain338/1  "IMAPve_d_EPB_Display_Req"
  Constant321/1 -> Switch159/2
  Constant320/1 -> Switch159/1
  SWINve_y_ESC_EPBDisplayMessageReq/1 -> Switch159/3
  Switch160/1 -> Gain339/1  "IMAPve_d_EPB_Warn_Req"
  Constant323/1 -> Switch160/2
  Constant322/1 -> Switch160/1
  SWINve_y_ESC_EPBWarningIndicationReq/1 -> Switch160/3
  Switch161/1 -> Gain340/1  "IMAPve_d_EPB_Switch_State"
  Constant325/1 -> Switch161/2
  Constant324/1 -> Switch161/1
  SWINve_y_ESC_EPBSwitchStatics/1 -> Switch161/3
  Switch162/1 -> Gain341/1  "IMAPve_d_EPB_Switch_Valid"
  Constant327/1 -> Switch162/2
  Constant326/1 -> Switch162/1
  SWINve_y_ESC_EPBSwitchStaticsValidity/1 -> Switch162/3
  Switch163/1 -> Gain86/1  "IMAPve_d_ESC_Drive_Direction"
  Constant329/1 -> Switch163/2
  Constant328/1 -> Switch163/1
  SWINve_y_Vehicle_driving_direction/1 -> Switch163/3
  Switch164/1 -> Gain87/1  "IMAPve_d_ESC_Hold_State"
  Constant331/1 -> Switch164/2
  Constant330/1 -> Switch164/1
  SWINve_y_Vehicle_Hold_Status/1 -> Switch164/3
  Switch165/1 -> Gain336/1  "IMAPve_d_ESC_EBD_AlarmSig"
  Constant333/1 -> Switch165/2
  Constant332/1 -> Switch165/1
  SWINve_y_ESC_EBDAlarmSig/1 -> Switch165/3
  Switch166/1 -> Gain337/1  "IMAPve_d_ESC_AVH_Status"
  Constant335/1 -> Switch166/2
  Constant334/1 -> Switch166/1
  SWINve_y_ESC_AVHStatus/1 -> Switch166/3
  Switch167/1 -> Gain84/1  "IMAPve_d_ESC_FLW_Direction"
  Constant337/1 -> Switch167/2
  Constant336/1 -> Switch167/1
  SWINve_y_ESC_FLWDirection/1 -> Switch167/3
  Switch168/1 -> Gain89/1  "IMAPve_d_ESC_FRW_Direction"
  Constant339/1 -> Switch168/2
  Constant338/1 -> Switch168/1
  SWINve_y_ESC_FRWDirection/1 -> Switch168/3
  Switch169/1 -> Gain90/1  "IMAPve_d_ESC_TCS_ErrorStatus"
  Constant341/1 -> Switch169/2
  Constant340/1 -> Switch169/1
  SWINve_y_ESC_TCSErrorStatus/1 -> Switch169/3
  Switch170/1 -> Gain91/1  "IMAPve_d_ESC_RLW_Direction"
  Constant343/1 -> Switch170/2
  Constant342/1 -> Switch170/1
  SWINve_y_ESC-RLWDirection/1 -> Switch170/3
  Switch171/1 -> Gain92/1  "IMAPve_d_ESC_RRW_Direction"
  Constant345/1 -> Switch171/2
  Constant344/1 -> Switch171/1
  SWINve_y_ESC_RRWDirection/1 -> Switch171/3
  Switch172/1 -> Gain93/1  "IMAPve_d_ESC_EPB_ErrorStatus"
  Constant347/1 -> Switch172/2
  Constant346/1 -> Switch172/1
  SWINve_y_ESC_EPBErrorStatus/1 -> Switch172/3
  Switch173/1 -> Gain442/1  "IMAPve_g_ESC_BrkWhlCylinder_Pressure"
  Constant349/1 -> Switch173/2
  Constant348/1 -> Switch173/1
  SWINve_g_ESC_BrakeWheelCylinderPressure/1 -> Switch173/3
  SDFAve_y_Radar_FaultBitSetting_Signal/1 -> Gain5/1
  Data Type Conversion9/1 -> Terminator16/1  "ob_IMAPve_d_Radar_FaultBitSetting_Signal"
  Gain5/1 -> Data Type Conversion9/1, IMAPve_d_Radar_FaultBitSetting_Signal/1  "IMAPve_d_Radar_FaultBitSetting_Signal"
  Constant354/1 -> Switch174/2
  Switch174/1 -> Gain95/1
